simulink library "tpm"  (R2021b)
settings: Solver=VariableStepAuto  StartTime=0.0  StopTime=10.0  RelTol=1e-3
undefined symbols (not defined in the file or in its folder): ENUM_AN_LF, ENUM_AN_LR, ENUM_AN_RF, ENUM_AN_RR, ENUM_POWERSTA_OFF, ENUM_POWERSTA_OFFA, ENUM_POWERSTA_OFFC, ENUM_POWERSTA_ON, ENUM_POWERSTA_READY, ENUM_POWERSTA_STANDBY, ENUM_PWRSTASW_OFF, ENUM_PWRSTASW_OFFA, ENUM_PWRSTASW_OFFCHVCHRG, ENUM_PWRSTASW_STANDBY, ENUM_TPMSSNESORIDREGSTA_START, FALSE, KTPM_DataInVehSpdThreshold_kph, KTPM_Delay_raw8, KTPM_DiagLearn_flg, KTPM_TPMSModelVersion_raw, KTPM_WhlRotDir_enum_ovrdflg, KTPM_WhlRotDir_enum_ovrdval, TRUE, ZERO_FLOAT, ZERO_INT
libraries: simulink x58, $bdroot x27, hcu_lib x24
(part 9 of 9)

== stateflow chart tpm/TPM/TPMS/TPMS/Learn/LowerTirePressureCalibration/WarningPressureLearn5 ==
  state WarningPressureLearn [parallel]
    settings: executionOrder=1
    state Standby
      en:
      C=0;
      P=0;
      T=0;
      VTPM_P2alarm_raw=93;
      SPressindi=0;
    state Status
      en:
      P=P+VINP_Pin_raw8;
      T=T+VINP_Tin_raw8;
      C=C+1;
      SPressindi=3;
    state Calculate
      en:
      Pavg=P>>2;
      Tavg=T>>2;
      Pavg20=(Pavg*1.72+151)*(273+20)/(273+Tavg)-101;
    state Nopass
      en:
      SPressindi=2;
    state Pass
      en:
      SPressindi=1;
      VTPM_P2alarm_raw=(Pavg20*0.8+14-50)/1.72;
    (default) -> Standby
    Status -> Standby [order 2] : [VINP_TPMSResButt_flg||VINP_TPMSCaliButt_flg||VTPM_S2timeout_flg]
    Status -> Calculate [order 1] : [C>=4]
    Standby -> (junction 217) : [VINP_DATAin_flg&&!VINP_TPMSResButt_flg&&(VTPM_IDLOCK_flg||VTPM_LocationDone_flg)]
    (junction 217) -> Status : [VINP_IDin_raw32==VTPM_S2ID_raw32....
        | &&VINP_Pin_raw8!=0&&VINP_Tin_raw8!=0]
    (junction 235) -> (junction 217)
    Status -> (junction 235) [order 3] : [VINP_DATAin_flg&&C<4]
    Nopass -> Standby : [VINP_TPMSResButt_flg||VINP_TPMSCaliButt_flg]
    (junction 69) -> Nopass [order 2]
    Calculate -> (junction 69)
    (junction 69) -> Pass [order 1] : [Pavg20>245]
    Pass -> Standby : [VINP_TPMSResButt_flg||VINP_TPMSCaliButt_flg]
  data: VINP_Pin_raw8 input; VINP_Tin_raw8 input; VINP_IDin_raw32 input; VINP_DATAin_flg input; VINP_TPMSResButt_flg input; VINP_TPMSCaliButt_flg input; VTPM_IDLOCK_flg input; VTPM_P2alarm_raw output uint8; Pavg20 local single; SPressindi output uint8; P local single; Pavg local single; T local single; Tavg local single; VTPM_S2ID_raw32 input; C local uint8; VTPM_LocationDone_flg input; VTPM_S2timeout_flg input

== stateflow chart tpm/TPM/TPMS/TPMS/Learn/LowerTirePressureCalibration/WarningPressureLearn ==
  state WarningPressureLearn
    state Initial
    state Calculate
      en:
      P=VTPM_ManualID1pressure_raw;
      T=VTPM_ManualID1Temp_C;
      Pavg20=(P*1.72+151)*(273+20)/(273+T)-101;
      VTPM_ManualID1P20_raw8=uint8(((double(P)*1.72+151)*(273+20)/(273+double(T))-151)/1.72);
    state Standby
      en:
      P=0;
      T=0;
      VTPM_P1alarm_raw=93;
      VTPM_S1pressindi_enum=0;
    state Nopass
      en:
      VTPM_S1pressindi_enum=2;
    state Pass
      en:
      VTPM_S1pressindi_enum=1;
      VTPM_P1alarm_raw=(Pavg20*0.8+14-50)/1.72;
    (default) -> Initial
    Initial -> Standby : [DiagLearn]
    Standby -> Calculate : [VTPM_TPMSmanualDone_flg]
    Calculate -> (junction 69)
    (junction 69) -> Nopass [order 2]
    Nopass -> Standby : [DiagLearn]
    (junction 69) -> Pass [order 1] : [Pavg20>245]
    Pass -> Standby : [DiagLearn]
  data: VTPM_ManualID1pressure_raw input; VTPM_ManualID1Temp_C input; VTPM_P1alarm_raw output uint8; Pavg20 local single; VTPM_S1pressindi_enum output uint8; P local single; T local single; DiagLearn input; VTPM_TPMSmanualDone_flg input boolean; VTPM_ManualID1P20_raw8 output uint8

== stateflow chart tpm/TPM/TPMS/TPMS/Learn/AutoLocation/WheelPosition/Chart1 ==
  state Start
    state Forward
      en:
      a=(VTPM_LFWpos_raw+Delta);
      b=(VTPM_LFWpos_raw+Delta)/96;
      VTPM_LFWpos_raw=a-b*96;
    state Else
    state Backward
      en:
      a=(VTPM_LFWpos_raw+Delta);
      b=(VTPM_LFWpos_raw+Delta)/96;
      VTPM_LFWpos_raw=a-b*96;
    (default) -> (junction 54) : {VTPM_LFWpos_raw=0; Delta=0; PulseCountBuf=VINP_LFPulseCount_cnt;}
    Start -> (junction 54) : [hasChanged(VINP_LFPulseCount_cnt)]....
        | {Delta=VINP_LFPulseCount_cnt-PulseCountBuf;
        | PulseCountBuf=VINP_LFPulseCount_cnt;}
    (junction 54) -> (junction 47) [order 1] : [VPMM_PowerSta_enum!=ENUM_PWRSTASW_OFF&&....
        |  VPMM_PowerSta_enum!=ENUM_PWRSTASW_OFFCHVCHRG&&...
        |  VPMM_PowerSta_enum!=ENUM_PWRSTASW_OFFA&&....
        |  VPMM_PowerSta_enum!=ENUM_PWRSTASW_STANDBY&&....
        |  VINP_LFPulseCountV_flg==false]
    (junction 47) -> (junction 6) [order 1] : [VTPM_LFWhlRotDir_enum==1]
    (junction 6) -> Forward [order 1] : [Delta>0]
    (junction 54) -> Else [order 2]
    (junction 47) -> (junction 48) [order 2]
    (junction 6) -> (junction 10) [order 2] : [Delta<0]
    (junction 10) -> Forward : {Delta=Delta+256;}
    (junction 48) -> Else [order 2]
    (junction 48) -> (junction 14) [order 1] : [VTPM_LFWhlRotDir_enum==2]
    (junction 14) -> Backward [order 1] : [Delta>0]{Delta=-Delta+96;}
    (junction 14) -> (junction 16) [order 2] : [Delta<0]
    (junction 16) -> Backward : {Delta=-Delta+128;}
  data: VPMM_PowerSta_enum input; VINP_LFPulseCount_cnt input; VINP_LFPulseCountV_flg input; VTPM_LFWhlRotDir_enum input; VTPM_LFWpos_raw output int16; a local int16; b local int16; Delta local int16; PulseCountBuf local int16; ENUM_PWRSTASW_OFF parameter; ENUM_PWRSTASW_OFFA parameter; ENUM_PWRSTASW_OFFCHVCHRG parameter; ENUM_PWRSTASW_STANDBY parameter

== stateflow chart tpm/TPM/TPMS/TPMS/Learn/LowerTirePressureCalibration/WarningPressureLearn2 ==
  state WarningPressureLearn
    state Initial
    state Calculate1
      en:
      P=VTPM_ManualID2pressure_raw;
      T=VTPM_ManualID2Temp_C;
      Pavg20=(P*1.72+151)*(273+20)/(273+T)-101;
      VTPM_ManualID2P20_raw8=uint8(((double(P)*1.72+151)*(273+20)/(273+double(T))-151)/1.72);
    state Standby
      en:
      P=0;
      T=0;
      VTPM_P2alarm_raw=93;
      VTPM_S2pressindi_enum=0;
    state Nopass
      en:
      VTPM_S2pressindi_enum=2;
    state Pass
      en:
      VTPM_S2pressindi_enum=1;
      VTPM_P2alarm_raw=(Pavg20*0.8+14-50)/1.72;
    (default) -> Initial
    Initial -> Standby : [DiagLearn]
    Standby -> Calculate1 : [VTPM_TPMSmanualDone_flg]
    Calculate1 -> (junction 69)
    (junction 69) -> Nopass [order 2]
    Nopass -> Standby : [DiagLearn]
    (junction 69) -> Pass [order 1] : [Pavg20>245]
    Pass -> Standby : [DiagLearn]
  data: VTPM_ManualID2pressure_raw input; VTPM_ManualID2Temp_C input; VTPM_P2alarm_raw output uint8; Pavg20 local single; VTPM_S2pressindi_enum output uint8; P local single; T local single; DiagLearn input; VTPM_TPMSmanualDone_flg input boolean; VTPM_ManualID2P20_raw8 output uint8

== stateflow chart tpm/TPM/TPMS/TPMS/Learn/LowerTirePressureCalibration/WarningPressureLearn6 ==
  state WarningPressureLearn
    state Initial
    state Calculate1
      en:
      P=VTPM_ManualID3pressure_raw;
      T=VTPM_ManualID3Temp_C;
      Pavg20=(P*1.72+151)*(273+20)/(273+T)-101;
      VTPM_ManualID3P20_raw8=uint8(((double(P)*1.72+151)*(273+20)/(273+double(T))-151)/1.72);
    state Standby
      en:
      P=0;
      T=0;
      VTPM_P3alarm_raw=93;
      VTPM_S3pressindi_enum=0;
    state Nopass
      en:
      VTPM_S3pressindi_enum=2;
    state Pass
      en:
      VTPM_S3pressindi_enum=1;
      VTPM_P3alarm_raw=(Pavg20*0.8+14-50)/1.72;
    (default) -> Initial
    Initial -> Standby : [DiagLearn]
    Standby -> Calculate1 : [VTPM_TPMSmanualDone_flg]
    Calculate1 -> (junction 69)
    (junction 69) -> Nopass [order 2]
    Nopass -> Standby : [DiagLearn]
    (junction 69) -> Pass [order 1] : [Pavg20>245]
    Pass -> Standby : [DiagLearn]
  data: VTPM_ManualID3pressure_raw input; VTPM_ManualID3Temp_C input; VTPM_P3alarm_raw output uint8; Pavg20 local single; VTPM_S3pressindi_enum output uint8; P local single; T local single; DiagLearn input; VTPM_TPMSmanualDone_flg input boolean; VTPM_ManualID3P20_raw8 output uint8

== stateflow chart tpm/TPM/TPMS/TPMS/Learn/LowerTirePressureCalibration/WarningPressureLearn7 ==
  state WarningPressureLearn
    state Initial
    state Status
      en:
      P=VTPM_ManualID4pressure_raw;
      T=VTPM_ManualID4Temp_C;
      Pavg20=(P*1.72+151)*(273+20)/(273+T)-101;
      VTPM_ManualID4P20_raw8=uint8(((double(P)*1.72+151)*(273+20)/(273+double(T))-151)/1.72);
    state Standby
      en:
      P=0;
      T=0;
      VTPM_P4alarm_raw=93;
      VTPM_S4pressindi_enum=0;
    state Nopass
      en:
      VTPM_S4pressindi_enum=2;
    state Pass
      en:
      VTPM_S4pressindi_enum=1;
      VTPM_P4alarm_raw=(Pavg20*0.8+14-50)/1.72;
    (default) -> Initial
    Initial -> Standby : [DiagLearn]
    Standby -> Status : [VTPM_TPMSmanualDone_flg]
    Status -> (junction 69)
    (junction 69) -> Nopass [order 2]
    Nopass -> Standby : [DiagLearn]
    (junction 69) -> Pass [order 1] : [Pavg20>245]
    Pass -> Standby : [DiagLearn]
  data: VTPM_ManualID4pressure_raw input; VTPM_ManualID4Temp_C input; VTPM_P4alarm_raw output uint8; Pavg20 local single; VTPM_S4pressindi_enum output uint8; P local single; T local single; DiagLearn input; VTPM_TPMSmanualDone_flg input boolean; VTPM_ManualID4P20_raw8 output uint8

== stateflow chart tpm/TPM/TPMS/TPMS/Learn/AutoLocation/Subsystem1/Subsystem/Chart ==
  state Manual
    (default) -> (junction 15) : {VTPM_TPMSStorge_flg=VINP_TPMSStorge_flg;
        | VTPM_MSensor1ID_raw=VINP_S1ID_raw;
        |  VTPM_MSensor2ID_raw=VINP_S2ID_raw;
        |  VTPM_MSensor3ID_raw=VINP_S3ID_raw;
        |  VTPM_MSensor4ID_raw=VINP_S4ID_raw;
        |  VTPM_MLFID_raw=VINP_LFID_raw;
        |  VTPM_MRFID_raw=VINP_RFID_raw;
        |  VTPM_MLRID_raw=VINP_LRID_raw;
        |  VTPM_MRRID_raw=VINP_RRID_raw;}
    Manual -> (junction 15) : [VINP_TPMSResButt_flg||VTPM_TPMSmanualDone_flg]
    (junction 15) -> (junction 17) [order 1] : [VTPM_TPMSmanualDone_flg]
    (junction 15) -> (junction 19) [order 2]
    (junction 17) -> (junction 21) : {VTPM_MSensor1ID_raw=VTPM_ManualID1_raw;
        |  VTPM_MSensor2ID_raw=VTPM_ManualID2_raw;
        |  VTPM_MSensor3ID_raw=VTPM_ManualID3_raw;
        |  VTPM_MSensor4ID_raw=VTPM_ManualID4_raw;
        |  VTPM_MLFID_raw=VTPM_ManualID1_raw;
        |  VTPM_MRFID_raw=VTPM_ManualID2_raw;
        |  VTPM_MLRID_raw=VTPM_ManualID3_raw
        |  VTPM_MRRID_raw=VTPM_ManualID4_raw;
        |  VTPM_TPMSStorge_flg=true;}
    (junction 19) -> (junction 23) [order 1] : [VINP_TPMSResButt_flg]
    (junction 19) -> (junction 27) [order 2]
    (junction 23) -> (junction 25) : {VTPM_MSensor1ID_raw=VINP_S1ID_raw;
        |  VTPM_MSensor2ID_raw=VINP_S2ID_raw;
        |  VTPM_MSensor3ID_raw=VINP_S3ID_raw;
        |  VTPM_MSensor4ID_raw=VINP_S4ID_raw;
        |  VTPM_MLFID_raw=VINP_LFID_raw;
        |  VTPM_MRFID_raw=VINP_RFID_raw;
        |  VTPM_MLRID_raw=VINP_LRID_raw;
        |  VTPM_MRRID_raw=VINP_RRID_raw;
        |  VTPM_TPMSStorge_flg=false;}
  data: VTPM_MSensor1ID_raw output; VTPM_MSensor2ID_raw output; VTPM_MSensor3ID_raw output; VTPM_MSensor4ID_raw output; VTPM_TPMSmanualDone_flg input; VINP_TPMSResButt_flg input; VINP_LFID_raw input; VINP_RFID_raw input; VINP_LRID_raw input; VINP_RRID_raw input; VTPM_ManualID1_raw input; VTPM_ManualID2_raw input; VTPM_ManualID3_raw input; VTPM_ManualID4_raw input; VTPM_TPMSStorge_flg output; VINP_S1ID_raw input; VINP_S2ID_raw input; VINP_S3ID_raw input; VINP_S4ID_raw input; VTPM_MLFID_raw output; VTPM_MLRID_raw output; VTPM_MRFID_raw output; VTPM_MRRID_raw output; VINP_TPMSStorge_flg input

== stateflow chart tpm/TPM/TPMS/TPMS/Learn/LowerTirePressureCalibration/WarningPressureLearn1 ==
  state WarningPressureLearn
    state Standby
      en:
      C=0;
      P=0;
      T=0;
      VTPM_P1alarm_raw=93;
      VTPM_S1pressindi_enum=0;
    state Status
      en:
      P=P+VINP_Pin_raw8;
      T=T+VINP_Tin_raw8;
      C=C+1;
      VTPM_S1pressindi_enum=3;
    state Calculate
      en:
      Pavg=P>>2;
      Tavg=T>>2;
      Pavg20=(Pavg*1.72+151)*(273+20)/(273+Tavg)-101;
    state Nopass
      en:
      VTPM_S1pressindi_enum=2;
    state Pass
      en:
      VTPM_S1pressindi_enum=1;
      VTPM_P1alarm_raw=(Pavg20*0.8+14-50)/1.72;
    (default) -> Standby
    Status -> Standby [order 2] : [VINP_TPMSResButt_flg||VINP_TPMSCaliButt_flg||VTPM_S1timeout_flg]
    Status -> Calculate [order 1] : [C>=4]
    Standby -> (junction 217) : [VINP_DATAin_flg&&!VINP_TPMSResButt_flg&&(VTPM_IDLOCK_flg||VTPM_LocationDone_flg)]
    (junction 217) -> Status : [VINP_IDin_raw32==VTPM_S1ID_raw32....
        | &&VINP_Pin_raw8!=0&&VINP_Tin_raw8!=0]
    (junction 235) -> (junction 217)
    Status -> (junction 235) [order 3] : [VINP_DATAin_flg&&C<4]
    (junction 69) -> Nopass [order 2]
    Calculate -> (junction 69)
    Nopass -> Standby : [VINP_TPMSResButt_flg||VINP_TPMSCaliButt_flg]
    (junction 69) -> Pass [order 1] : [Pavg20>245]
    Pass -> Standby : [VINP_TPMSResButt_flg||VINP_TPMSCaliButt_flg]
  data: VINP_Pin_raw8 input; VINP_Tin_raw8 input; VINP_IDin_raw32 input; VINP_DATAin_flg input; VINP_TPMSResButt_flg input; VINP_TPMSCaliButt_flg input; VTPM_IDLOCK_flg input; VTPM_P1alarm_raw output uint8; Pavg20 local single; VTPM_S1pressindi_enum output uint8; P local single; Pavg local single; T local single; Tavg local single; VTPM_S1ID_raw32 input; C output uint8; VTPM_S1timeout_flg input; VTPM_LocationDone_flg input

== stateflow chart tpm/TPM/TPMS/TPMS/Learn/AutoLocation/IDIdentify/Subsystem7/Chart ==
  state Sample [parallel]
    settings: executionOrder=1
    state DataNotEnough
    state Regisiter
      en:
      C=C+1;
      LFM=LF_PC;
      RFM=RF_PC;
      LRM=LR_PC;
      RRM=RR_PC;
    (default) -> DataNotEnough : {C=0;}
    DataNotEnough -> Regisiter [order 2] : [!VINP_TPMSResButt_flg&&GS]
    Regisiter -> (junction 513) [order 2] : [GS]
    (junction 513) -> (junction 514)
    (junction 514) -> Regisiter
    Regisiter -> DataNotEnough [order 1] : [VINP_TPMSResButt_flg]{C=0;}
    Regisiter -> (junction 528) [order 3] : [VPMM_PowerSta_enum!=ENUM_POWERSTA_ON&&...
        | VPMM_PowerSta_enum!=ENUM_POWERSTA_READY
        | ]
    (junction 528) -> (junction 532) : {C=0;}
    (junction 532) -> DataNotEnough
    DataNotEnough -> DataNotEnough [order 1] : [VINP_TPMSResButt_flg]{C=0;}
  data: VINP_TPMSResButt_flg input; VPMM_PowerSta_enum input; GS input; LR_PC input; LF_PC input; RR_PC input; RF_PC input; LFM output int16; LRM output int16; RRM output int16; RFM output int16; C output uint8; ENUM_POWERSTA_READY parameter; ENUM_POWERSTA_ON parameter

== matlab function tpm/TPM/TPMS/TPMS/Learn/LowerTirePressureCalibration/LPindSwitch ==
  data: LFP output; P1 input; P2 input; P3 input; P4 input; S1L input; S2L input; S3L input; S4L input; RFP output; LRP output; RRP output
function [LFP,RFP,LRP,RRP] = fcn(P1,P2,P3,P4,S1L,S2L,S3L,S4L)
P=[P1 P2 P3 P4];
S=[S1L S2L S3L S4L];
LFP=uint8(0);
RFP=uint8(0);
LRP=uint8(0);
RRP=uint8(0);
for i=1:length(S)
    if S(i)==1
        LFP=uint8(P(i));
    elseif S(i)==2
        RFP=uint8(P(i));
    elseif S(i)==3
        LRP=uint8(P(i));
    elseif S(i)==4
        RRP=uint8(P(i));
    end
end

== matlab function tpm/TPM/TPMS/TPMS/Learn/LowerTirePressureCalibration/LPindSwitch1 ==
  data: LFP output; P1 input; P2 input; P3 input; P4 input; S1L input; S2L input; S3L input; S4L input; RFP output; LRP output; RRP output
function [LFP,RFP,LRP,RRP] = fcn(P1,P2,P3,P4,S1L,S2L,S3L,S4L)
P=[P1 P2 P3 P4];
S=[S1L S2L S3L S4L];
LFP=uint8(0);
RFP=uint8(0);
LRP=uint8(0);
RRP=uint8(0);
for i=1:length(S)
    if S(i)==1
        LFP=uint8(P(i));
    elseif S(i)==2
        RFP=uint8(P(i));
    elseif S(i)==3
        LRP=uint8(P(i));
    elseif S(i)==4
        RRP=uint8(P(i));
    end
end

== stateflow chart tpm/TPM/TPMS/TPMS/Send/DATA/LocationSW/Chart1 ==
  state Location [parallel]
    settings: executionOrder=1
    state S1
      en:SLocation=VTPM_S1L_enum;
    state S2
      en:SLocation=VTPM_S2L_enum;
    state S3
      en:SLocation=VTPM_S3L_enum;
    state S4
      en:SLocation=VTPM_S4L_enum;
    state Else
      en:SLocation=0;
    (default) -> (junction 72)
    (junction 6) -> S1 [order 1] : [VTPM_IDLOCK_flg && VINP_DATAin_flg && VINP_IDin_raw32==VTPM_S1ID_raw32]
    Location -> (junction 72)
    (junction 72) -> (junction 6) [order 1] : [VPMM_PowerSta_enum==ENUM_POWERSTA_ON||...
        | VPMM_PowerSta_enum==ENUM_POWERSTA_READY]
    (junction 72) -> Location.Else [order 2]
    (junction 6) -> (junction 7) [order 2]
    (junction 7) -> S2 [order 1] : [VTPM_IDLOCK_flg && VINP_DATAin_flg && VINP_IDin_raw32==VTPM_S2ID_raw32]
    (junction 7) -> (junction 10) [order 2]
    (junction 10) -> S3 [order 1] : [VTPM_IDLOCK_flg && VINP_DATAin_flg && VINP_IDin_raw32==VTPM_S3ID_raw32]
    (junction 10) -> (junction 1) [order 2]
    (junction 1) -> S4 [order 1] : [VTPM_IDLOCK_flg && VINP_DATAin_flg && VINP_IDin_raw32==VTPM_S4ID_raw32]
    (junction 1) -> Location.Else [order 2]
  state Identify [parallel]
    settings: executionOrder=2
    state LF
      en:VTPM_LFSW_flg=true;VTPM_RFSW_flg=false;VTPM_LRSW_flg=false;VTPM_RRSW_flg=false;
    state RF
      en:VTPM_LFSW_flg=false;VTPM_RFSW_flg=true;VTPM_LRSW_flg=false;VTPM_RRSW_flg=false;
    state LR
      en:VTPM_LFSW_flg=false;VTPM_RFSW_flg=false;VTPM_LRSW_flg=true;VTPM_RRSW_flg=false;
    state RR
      en:VTPM_LFSW_flg=false;VTPM_RFSW_flg=false;VTPM_LRSW_flg=false;VTPM_RRSW_flg=true;
    state Else
      en:VTPM_LFSW_flg=false;VTPM_RFSW_flg=false;VTPM_LRSW_flg=false;VTPM_RRSW_flg=false;
    (default) -> (junction 42)
    Identify -> (junction 42)
    (junction 42) -> LF [order 1] : [SLocation==ENUM_AN_LF]
    (junction 42) -> (junction 46) [order 2]
    (junction 46) -> RF [order 1] : [SLocation==ENUM_AN_RF]
    (junction 46) -> (junction 56) [order 2]
    (junction 56) -> LR [order 1] : [SLocation==ENUM_AN_LR]
    (junction 56) -> (junction 47) [order 2]
    (junction 47) -> RR [order 1] : [SLocation==ENUM_AN_RR]
    (junction 47) -> Identify.Else [order 2]
  data: VTPM_S1ID_raw32 input; VPMM_PowerSta_enum input; VTPM_S1L_enum input; VTPM_S2ID_raw32 input; VTPM_S2L_enum input; VTPM_S3ID_raw32 input; VTPM_S3L_enum input; VTPM_S4ID_raw32 input; VTPM_S4L_enum input; VINP_IDin_raw32 input; VINP_DATAin_flg input; VTPM_IDLOCK_flg input; VTPM_LFSW_flg output boolean; VTPM_RFSW_flg output boolean; VTPM_LRSW_flg output boolean; VTPM_RRSW_flg output boolean; SLocation local uint8; ENUM_AN_LF parameter; ENUM_AN_LR parameter; ENUM_AN_RF parameter; ENUM_AN_RR parameter; ENUM_POWERSTA_ON parameter; ENUM_POWERSTA_READY parameter

== matlab function tpm/TPM/TPMS/TPMS/Learn/AutoLocation/Doublecheck/MATLAB Function ==
  data: S1ID input; LFID output; S2ID input; S3ID input; S4ID input; S1L input; S2L input; S3L input; S4L input; VTPM_ALLFin_flg input; RFID output; LRID output; RRID output
function [LFID, RFID, LRID, RRID] = fcn(S1ID, S2ID, S3ID, S4ID, S1L, S2L, S3L, S4L, VTPM_ALLFin_flg)
    LFID = uint32(0);
    RFID = uint32(0);
    LRID = uint32(0);
    RRID = uint32(0);
    
    if VTPM_ALLFin_flg == 1
        ID = [S1ID, S2ID, S3ID, S4ID];
        Location = [S1L, S2L, S3L, S4L];
        
        for i = 1:length(Location)
            if Location(i) == 1
                LFID = uint32(ID(i));
            elseif Location(i) == 2
                RFID = uint32(ID(i));
            elseif Location(i) == 3
                LRID = uint32(ID(i));
            elseif Location(i) == 4
                RRID = uint32(ID(i));
            end
        end
    end
end

== stateflow chart tpm/TPM/TPMS/TPMS/Subsystem/Chart ==
  state WriteChkLFID [parallel]
    settings: executionOrder=1
    (default) -> (junction 131)
    WriteChkLFID -> (junction 131) : [VTPM_SetChkId_flg||VINP_TPMSResButt_flg]
    (junction 131) -> (junction 102) : {
        | VTPM_WriteChkLFID_raw=VTPM_WriteLFID_raw;
        | VTPM_WriteChkRFID_raw=VTPM_WriteRFID_raw;
        | VTPM_WriteChkLRID_raw=VTPM_WriteLRID_raw;
        | VTPM_WriteChkRRID_raw=VTPM_WriteRRID_raw;
        | VTPM_Flashchkdatavalid_flg=1;
        | }
    (junction 102) -> (junction 104) [order 1] : [VINP_TPMSResButt_flg||!VTPM_SetChkId_flg]
    (junction 102) -> (junction 108) [order 2]
    (junction 104) -> (junction 106) : {VTPM_WriteChkLFID_raw=ZERO_INT;
        | VTPM_WriteChkRFID_raw=ZERO_INT;
        | VTPM_WriteChkLRID_raw=ZERO_INT;
        | VTPM_WriteChkRRID_raw=ZERO_INT;
        | VTPM_Flashchkdatavalid_flg=0;
        | }
    (junction 106) -> (junction 108)
  state WriteChkFinLFID [parallel]
    settings: executionOrder=2
    (default) -> (junction 128)
    WriteChkFinLFID -> (junction 128) : [VTPM_CheckFin_flg||VINP_TPMSResButt_flg]
    (junction 128) -> (junction 112) : {VTPM_WriteChkfinLFID_raw=VTPM_WriteLFID_raw;
        | VTPM_WriteChkfinRFID_raw=VTPM_WriteRFID_raw;
        | VTPM_WriteChkfinLRID_raw=VTPM_WriteLRID_raw;
        | VTPM_WriteChkfinRRID_raw=VTPM_WriteRRID_raw;
        | VTPM_Flashdatavalid_flg=1;
        | }
    (junction 112) -> (junction 113) [order 1] : [VINP_TPMSResButt_flg||!VTPM_CheckFin_flg]
    (junction 112) -> (junction 116) [order 2]
    (junction 113) -> (junction 114) : {
        | VTPM_WriteChkfinLFID_raw=ZERO_INT;
        | VTPM_WriteChkfinRFID_raw=ZERO_INT;
        | VTPM_WriteChkfinLRID_raw=ZERO_INT;
        | VTPM_WriteChkfinRRID_raw=ZERO_INT;
        | VTPM_Flashdatavalid_flg=0;
        | }
    (junction 114) -> (junction 116)
  data: VTPM_WriteLFID_raw input; VTPM_WriteRFID_raw input; VTPM_WriteLRID_raw input; VTPM_WriteRRID_raw input; ZERO_INT parameter; VTPM_CheckFin_flg input; VTPM_WriteChkLFID_raw output uint32; VTPM_WriteChkLRID_raw output uint32; VTPM_WriteChkRFID_raw output uint32; VTPM_WriteChkRRID_raw output uint32; VTPM_WriteChkfinLFID_raw output uint32; VTPM_WriteChkfinLRID_raw output uint32; VTPM_WriteChkfinRFID_raw output uint32; VTPM_WriteChkfinRRID_raw output uint32; VINP_TPMSResButt_flg input; VTPM_SetChkId_flg input; VTPM_Flashchkdatavalid_flg output boolean; VTPM_Flashdatavalid_flg output boolean

== matlab function tpm/TPM/TPMS/TPMS/Subsystem/MATLAB Function ==
  data: S1ID input; LFID output; S2ID input; S3ID input; S4ID input; S1L input; S2L input; S3L input; S4L input; set input; RFID output; LRID output; RRID output
function [LFID, RFID, LRID, RRID] = fcn(S1ID, S2ID, S3ID, S4ID, S1L, S2L, S3L, S4L, set)
    LFID = uint32(0);
    RFID = uint32(0);
    LRID = uint32(0);
    RRID = uint32(0);
    
    if set == 1
        ID = [S1ID, S2ID, S3ID, S4ID];
        Location = [S1L, S2L, S3L, S4L];
        
        for i = 1:length(Location)
            if Location(i) == 1
                LFID = uint32(ID(i));
            elseif Location(i) == 2
                RFID = uint32(ID(i));
            elseif Location(i) == 3
                LRID = uint32(ID(i));
            elseif Location(i) == 4
                RRID = uint32(ID(i));
            end
        end
    end
end
